simulink model "test_cg_1"  (R2022b)
settings: Solver=FixedStepAuto  StartTime=0.0  StopTime=10.0  FixedStep=1e-3  RelTol=1e-3
settings Model: Creator=asolland  LastModifiedBy=asolland
settings OptimizationCC: DefaultParameterBehavior=Inlined  EnhancedBackFolding=on  PassReuseOutputArgsAs=Individual arguments  OptimizeBlockOrder=speed  DifferentSizesBufferReuse=on  OptimizationCustomize=off  EfficientTunableParamExpr=on
settings DebuggingCC: ParameterTunabilityLossMsg=error
settings HardwareCC: TargetBitPerLong=64  TargetBitPerPointer=64  TargetBitPerSizeT=64  TargetBitPerPtrDiffT=64  TargetLongLongMode=on  TargetIntDivRoundTo=Zero  TargetEndianess=LittleEndian  TargetWordSize=64  TargetHWDeviceType=MATLAB Host  ProdEqTarget=off
settings SFSimCC: MATLABDynamicMemAlloc=off
settings RTWCC: Description=Embedded Coder (host-based shared library target)  SystemTargetFile=sim_pandas.tlc  TemplateMakefile=ert_default_tmf  GPUComputeCapability=5.0
settings CodeAppCC: ForceParamTrailComments=on  IgnoreCustomStorageClasses=off  OperatorAnnotations=on  SimulinkDataObjDesc=on  SFDataObjDesc=on  InsertBlockDesc=on
settings STFCustomTargetCC: TargetLangStandard=C99 (ISO)  MultiwordLength=256  GenerateSampleERTMain=on  ParMdlRefBuildCompliant=on  CompOptLevelCompliant=on  CombineOutputUpdateFcns=on  ERTCustomFileBanners=on  CodeInterfacePackaging=Reusable function  SupportContinuousTime=off  SupportNonInlinedSFcns=off  RemoveResetFunc=on  MATLABClassNameForMDSCustomization=Simulink.SoftwareTarget.ERTCustomization  ModelStepFunctionPrototypeControlCompliant=on  UseToolchainInfoCompliant=on  SystemTargetFile=sim_pandas.tlc
settings ERTTargetCC: TargetLangStandard=C99 (ISO)  GenerateSampleERTMain=on  ConcurrentExecutionCompliant=off  CodeInterfacePackaging=Reusable function  CPPClassGenCompliant=off  InlinedParameterPlacement=NonHierarchical  RootIOFormat=Part of model data structure  ERTCustomFileTemplate=example_file_process.tlc

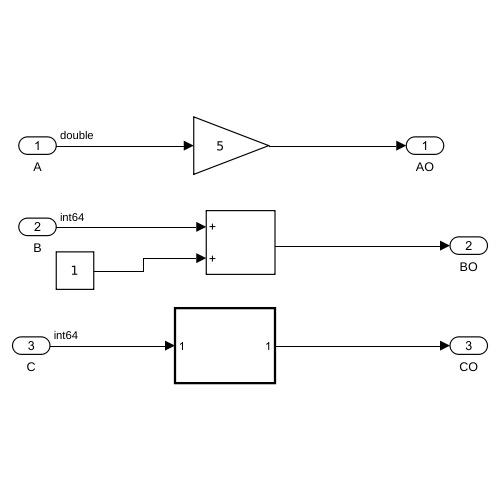
[thumbnail: Simulink's stored preview of the top-level diagram]
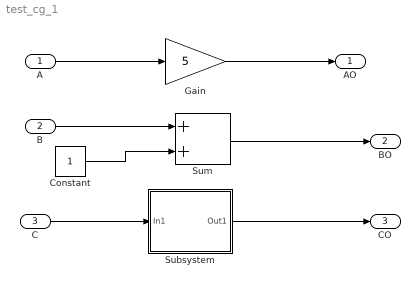
== system test_cg_1 ==
  A : Inport  OutDataTypeStr=double
  B : Inport  Port=2  OutDataTypeStr=int64
  C : Inport  Port=3  OutDataTypeStr=int64
  Constant : Constant  OutDataTypeStr=int64
  Gain : Gain  Gain=5
  Subsystem : Subsystem  TreatAsAtomicUnit=on
  Sum : Sum
  AO : Outport
  BO : Outport  Port=2
  CO : Outport  Port=3
  wires:
  A/1 -> Gain/1
  B/1 -> Sum/1
  Sum/1 -> BO/1
  Constant/1 -> Sum/2
  Gain/1 -> AO/1
  C/1 -> Subsystem/1(In1)
  Subsystem/1(Out1) -> CO/1

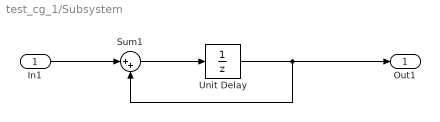
== system test_cg_1/Subsystem ==
  In1 : Inport
  Sum1 : Sum  Inputs=|++
  Unit Delay : UnitDelay  SampleTime=-1  HasFrameUpgradeWarning=on
  Out1 : Outport
  wires:
  Sum1/1 -> Unit Delay/1
  In1/1 -> Sum1/1
  Unit Delay/1 -> Out1/1, Sum1/2
